simulink model "SRF_PLL"  (R2025a)
settings: Solver=VariableStepAuto  StartTime=0.0  StopTime=0.12  RelTol=1e-3
libraries: spsSeriesRLCBranchLib x6, spsACVoltageSourceLib x3, spsVoltageMeasurementLib x3, sps_lib x1
settings Model: Creator=jicai  LastModifiedBy=jicai

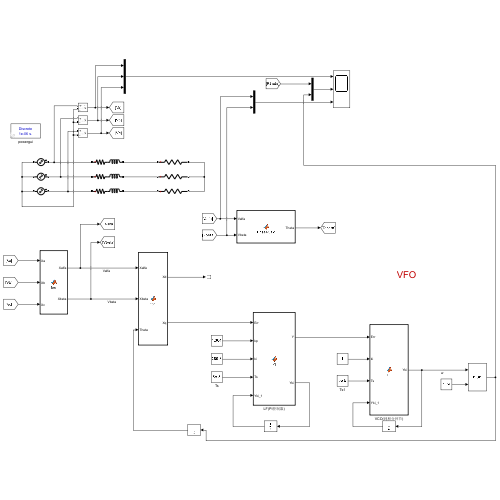
[thumbnail: Simulink's stored preview of the top-level diagram]
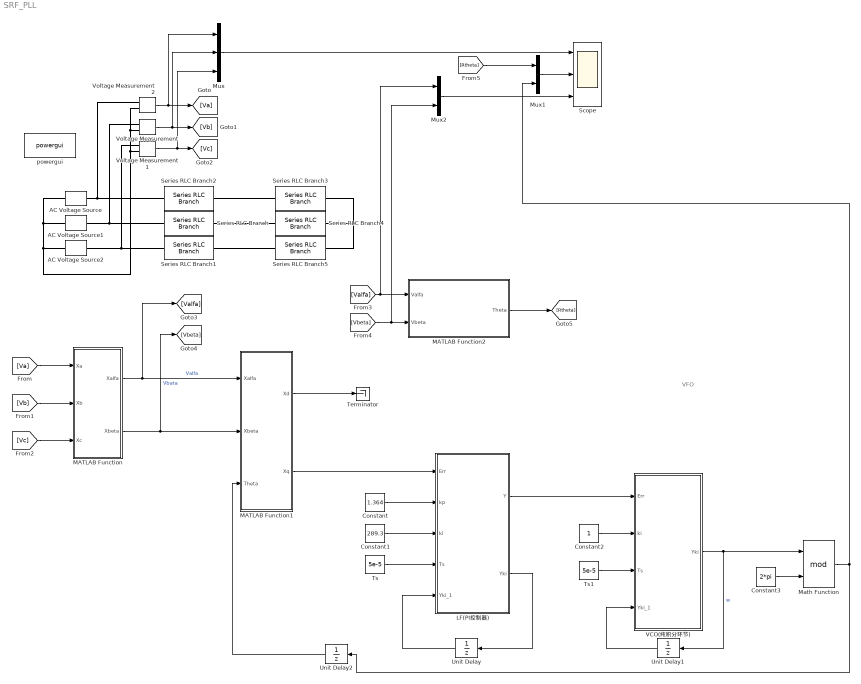
== system SRF_PLL ==
  note: VFO
  AC Voltage Source : spsACVoltageSourceLib/AC Voltage Source  Amplitude=220  Phase=-120  Frequency=50  SampleTime=0  Measurements=None  BusType=swing  Pref=10e3  Qref=0  Qmin=-inf  Qmax=+inf
  AC Voltage Source1 : spsACVoltageSourceLib/AC Voltage Source  Amplitude=220  Phase=0  Frequency=50  SampleTime=0  Measurements=None  BusType=swing  Pref=10e3  Qref=0  Qmin=-inf  Qmax=+inf
  AC Voltage Source2 : spsACVoltageSourceLib/AC Voltage Source  Amplitude=220  Phase=120  Frequency=50  SampleTime=0  Measurements=None  BusType=swing  Pref=10e3  Qref=0  Qmin=-inf  Qmax=+inf
  Constant : Constant  Value=1.364
  Constant1 : Constant  Value=289.3
  Constant2 : Constant
  Constant3 : Constant  Value=2*pi
  LF(PI控制器) : MATLAB Function  TreatAsAtomicUnit=on
  MATLAB Function : MATLAB Function  TreatAsAtomicUnit=on
  MATLAB Function1 : MATLAB Function  TreatAsAtomicUnit=on
  MATLAB Function2 : MATLAB Function  TreatAsAtomicUnit=on
  Math Function : Math  Operator=mod
  Mux : Mux  Inputs=3
  Mux1 : Mux  Inputs=2
  Mux2 : Mux  Inputs=2
  Scope : Scope  NumInputPorts=3
      settings: ActiveDisplayYMinimum=-275  ActiveDisplayYMaximum=275
  Series RLC Branch : spsSeriesRLCBranchLib/Series RLC Branch  LConnTagsString=__new0  RConnTagsString=__new0  BranchType=RL  Resistance=0.1  Inductance=1e-3  SetiL0=off  InitialCurrent=0  Capacitance=1e-6  Setx0=off  InitialVoltage=0  Measurements=None
  Series RLC Branch1 : spsSeriesRLCBranchLib/Series RLC Branch  LConnTagsString=__new0  RConnTagsString=__new0  BranchType=RL  Resistance=0.1  Inductance=1e-3  SetiL0=off  InitialCurrent=0  Capacitance=1e-6  Setx0=off  InitialVoltage=0  Measurements=None
  Series RLC Branch2 : spsSeriesRLCBranchLib/Series RLC Branch  LConnTagsString=__new0  RConnTagsString=__new0  BranchType=RL  Resistance=0.1  Inductance=1e-3  SetiL0=off  InitialCurrent=0  Capacitance=1e-6  Setx0=off  InitialVoltage=0  Measurements=None
  Series RLC Branch3 : spsSeriesRLCBranchLib/Series RLC Branch  LConnTagsString=__new0  RConnTagsString=__new0  BranchType=R  Resistance=100  Inductance=1e-3  SetiL0=off  InitialCurrent=0  Capacitance=1e-6  Setx0=off  InitialVoltage=0  Measurements=None
  Series RLC Branch4 : spsSeriesRLCBranchLib/Series RLC Branch  LConnTagsString=__new0  RConnTagsString=__new0  BranchType=R  Resistance=100  Inductance=1e-3  SetiL0=off  InitialCurrent=0  Capacitance=1e-6  Setx0=off  InitialVoltage=0  Measurements=None
  Series RLC Branch5 : spsSeriesRLCBranchLib/Series RLC Branch  LConnTagsString=__new0  RConnTagsString=__new0  BranchType=R  Resistance=100  Inductance=1e-3  SetiL0=off  InitialCurrent=0  Capacitance=1e-6  Setx0=off  InitialVoltage=0  Measurements=None
  Terminator : Terminator
  Ts : Constant  Value=5e-5
  Ts1 : Constant  Value=5e-5
  Unit Delay : UnitDelay  SampleTime=-1  HasFrameUpgradeWarning=on
  Unit Delay1 : UnitDelay  SampleTime=-1  HasFrameUpgradeWarning=on
  Unit Delay2 : UnitDelay  SampleTime=-1  HasFrameUpgradeWarning=on
  VCO(纯积分环节) : MATLAB Function  TreatAsAtomicUnit=on
  Voltage Measurement : spsVoltageMeasurementLib/Voltage Measurement  PhasorSimulation=off  OutputType=Complex  PSBequivalent=0
  Voltage Measurement1 : spsVoltageMeasurementLib/Voltage Measurement  PhasorSimulation=off  OutputType=Complex  PSBequivalent=0
  Voltage Measurement2 : spsVoltageMeasurementLib/Voltage Measurement  PhasorSimulation=off  OutputType=Complex  PSBequivalent=0
  powergui : sps_lib/powergui  Priority=1  SimulationMode=Discrete  SampleTime=1e-6  frequency=60  Iterations=50  frequencyindice=50  Pbase=100e6  ErrMax=1e-4  UnitsV=kV  UnitsW=MW  buscounter=0  FunctionMessages=off  echomessages=off  EnableUseOfTLC=off  CurrentSourceSwitches=off  DisableSnubberDevices=off  DisableRonSwitches=off  DisableVfSwitches=off  DisplayEquations=off  AutomaticDiscreteSolvers=off  SolverType=Tustin/Backward Euler (TBE)  Interpol=off  ExternalGateDelay=off  methode=off  Ts=100  x0status=blocks  SPID=on  SwTol=0  HookPort=off  NonlinearTolerance=1e-4  nMaxIteration=100  ContinueOnMaxIteration=off  RestoreLinks=warning  ResistiveCurrentMeasurement=off  Frange=[0:2:500]  Ylog=off  Xlog=on  ShowGrid=off  save=off  variable=ZData  structure=0  ZoomFFT=off  StartTime=0.0  cycles=1  DisplayStyle=1  fundamental=60  FreqAxis=off  MaxFrequency=1000  frequencyindicesteady=1  RmsSteady=1  display=off
  wires:
  Voltage Measurement2/1 -> Mux/1, [Va]
  Voltage Measurement/1 -> Mux/2, [Vb]
  Voltage Measurement1/1 -> Mux/3, [Vc]
  Mux/1 -> Scope/1
  [Va] -> MATLAB Function/1(Xa)
  [Vb] -> MATLAB Function/2(Xb)
  [Vc] -> MATLAB Function/3(Xc)
  MATLAB Function/1(Xalfa) -> [Valfa], MATLAB Function1/1(Xalfa)  "Valfa"
  MATLAB Function/2(Xbeta) -> [Vbeta], MATLAB Function1/2(Xbeta)  "Vbata"
  [Valfa] -> Mux2/1, MATLAB Function2/1(Valfa)
  [Vbeta] -> Mux2/2, MATLAB Function2/2(Vbeta)
  MATLAB Function2/1(Theta) -> [Rtheta]
  MATLAB Function1/2(Xq) -> LF(PI控制器)/1(Err)
  Constant/1 -> LF(PI控制器)/2(kp)
  Constant1/1 -> LF(PI控制器)/3(ki)
  Ts/1 -> LF(PI控制器)/4(Ts)
  LF(PI控制器)/2(Yki) -> Unit Delay/1
  Unit Delay/1 -> LF(PI控制器)/5(Yki_1)
  MATLAB Function1/1(Xd) -> Terminator/1
  LF(PI控制器)/1(Y) -> VCO(纯积分环节)/1(Err)
  Constant2/1 -> VCO(纯积分环节)/2(ki)
  Ts1/1 -> VCO(纯积分环节)/3(Ts)
  Unit Delay1/1 -> VCO(纯积分环节)/4(Yki_1)
  VCO(纯积分环节)/1(Yki) -> Unit Delay1/1, Math Function/1  "w"
  Constant3/1 -> Math Function/2
  Unit Delay2/1 -> MATLAB Function1/3(Theta)
  Math Function/1 -> Mux1/2, Unit Delay2/1
  [Rtheta] -> Mux1/1
  Mux1/1 -> Scope/2
  Mux2/1 -> Scope/3
  connections:
  Series RLC Branch2/LConn1 -- Voltage Measurement2/LConn1 -- AC Voltage Source/RConn1
  AC Voltage Source1/RConn1 -- Voltage Measurement/LConn1 -- Series RLC Branch/LConn1
  Series RLC Branch1/LConn1 -- Voltage Measurement1/LConn1 -- AC Voltage Source2/RConn1
  Series RLC Branch2/RConn1 -- Series RLC Branch3/LConn1
  Series RLC Branch/RConn1 -- Series RLC Branch4/LConn1
  Series RLC Branch1/RConn1 -- Series RLC Branch5/LConn1
  Series RLC Branch3/RConn1 -- Series RLC Branch4/RConn1 -- Series RLC Branch5/RConn1
  AC Voltage Source/LConn1 -- Voltage Measurement/LConn2 -- Voltage Measurement2/LConn2 -- Voltage Measurement1/LConn2 -- AC Voltage Source2/LConn1 -- AC Voltage Source1/LConn1

== matlab function SRF_PLL/MATLAB Function1 ==
  data: Xalfa input; Xd output; Xbeta input; Theta input; Xq output
function [Xd,Xq] = fcn(Xalfa,Xbeta,Theta)
Xd = Xalfa * cos(Theta) + Xbeta * sin(Theta);
Xq = -Xalfa * sin(Theta) + Xbeta * cos(Theta);

== matlab function SRF_PLL/MATLAB Function ==
  data: Xa input; Xalfa output; Xb input; Xc input; Xbeta output
function [Xalfa,Xbeta] = fcn(Xa,Xb,Xc)
Xalfa = 2/3*(Xa - 0.5*Xb - 0.5*Xc);
Xbeta = sqrt(3)/3*(Xb-Xc);

== matlab function SRF_PLL/MATLAB Function2 ==
  data: Valfa input; Theta output; Vbeta input
function Theta  = PhaseCalc(Valfa,Vbeta)
Theta = atan2(Vbeta,Valfa);
if Theta < 0
    Theta = Theta + 2*pi;
end
end

== matlab function SRF_PLL/LF(PI控制器) ==
  data: Err input; Y output; kp input; ki input; Yki output; Ts input; Yki_1 input
function [Y, Yki] = PI(Err, kp, ki,Ts,Yki_1)

% 采用的离散化方法： s = (1-z^{-1})/Ts

max = 3000;  % 限幅
min = -3000;

% 计算积分项
Yki = Yki_1 + Ts*ki*Err;
if Yki > max
    Yki = max;
elseif Yki < min
    Yki = min;
end

% 加上比例项 
Y = kp*Err + Yki;

if Y > max
    Y = max;
elseif Y < min
    Y = min;
end
end

== matlab function SRF_PLL/VCO(纯积分环节) ==
  data: Err input; ki input; Yki output; Ts input; Yki_1 input
function Yki  = PI(Err, ki,Ts,Yki_1)

% 采用的离散化方法： s = (1-z^{-1})/Ts

max = 3000;
min = -3000;

% 计算积分项
Yki = Yki_1 + Ts*ki*Err;

if Yki > max
    Yki = max;
elseif Yki < min
    Yki = min;
end
end
